simulink model "MotionObjectDetector"  (Simulink 10.0)
settings: Solver=FixedStepAuto  StartTime=0.0  StopTime=inf  RelTol=1e-3  EnableMultiTasking=on
undefined symbols (not defined in the file or in its folder): gray, Horn, hot, iut_dim, Kanade, Lucas, none, num_targets, pfactor, Rec, Schunck, SDTV, strel, target_dim, target_dim_nopyramid, videoinput
libraries: visionsinks x10, visionmorphops x7, visionanalysis x6, visionstatistics x5, visiontransforms x5, visiontextngfix x4, visionconversions x4, dspvision x3, visiongeotforms x2, visionutilities x2, imaqlib x1, visionsources x1
(part 1 of 2)
settings Model: Creator=fredd  LastModifiedBy=fredd  SimulationMode=accelerator  OrderedModelArguments=off
settings SolverCC: PositivePriorityOrder=on  AutoInsertRateTranBlk=on
settings DataIOCC: SaveFormat=Dataset  ReturnWorkspaceOutputs=on
settings OptimizationCC: DefaultParameterBehavior=Inlined  EnhancedBackFolding=on  PassReuseOutputArgsAs=Individual arguments  ZeroExternalMemoryAtStartup=off  ZeroInternalMemoryAtStartup=off  LifeSpan=auto  MaxStackSize=64  OptimizeBlockOrder=speed  DifferentSizesBufferReuse=on  OptimizationCustomize=off  EfficientTunableParamExpr=on
settings DebuggingCC: UnderspecifiedInitializationDetection=Simplified  MergeDetectMultiDrivingBlocksExec=error  ParameterTunabilityLossMsg=error  SFUnexpectedBacktrackingDiag=error  SFNoUnconditionalDefaultTransitionDiag=error  SFExecutionAtInitializationDiag=warning  ArithmeticOperatorsInVariantConditions=error
settings HardwareCC: ProdLargestAtomicInteger=Long  ProdLargestAtomicFloat=Double  ProdIntDivRoundTo=Zero  ProdEndianess=LittleEndian  ProdLongLongMode=on  ProdHWDeviceType=ARM Compatible->ARM Cortex
settings ModelReferenceCC: PropagateSignalLabelsOutOfModel=on
settings SFSimCC: SimUseLocalCustomCode=on  CustomCodeUndefinedFunction=FilterOut
settings RTWCC: Description=Embedded Coder  SystemTargetFile=ert.tlc  TemplateMakefile=ert_default_tmf  GenerateReport=on  RTWUseLocalCustomCode=on  Toolchain=GNU GCC Raspberry Pi  BuildConfiguration=Faster Runs  IncludeHyperlinkInReport=on  LaunchReport=on  GenerateTraceInfo=on  GenerateTraceReport=on  GenerateTraceReportSl=on  GenerateTraceReportSf=on  GenerateTraceReportEml=on
settings CodeAppCC: ForceParamTrailComments=on  IgnoreCustomStorageClasses=off  OperatorAnnotations=on  SimulinkDataObjDesc=on  SFDataObjDesc=on  InsertBlockDesc=on  StateflowObjectComments=off
settings ERTTargetCC: SupportVariableSizeSignals=on  ERTCustomFileTemplate=example_file_process.tlc
settings ConfigComp: CovMetricSettings=dwe  CovHtmlReporting=off  CovSaveCumulativeToWorkspaceVar=off  CovSaveSingleToWorkspaceVar=off

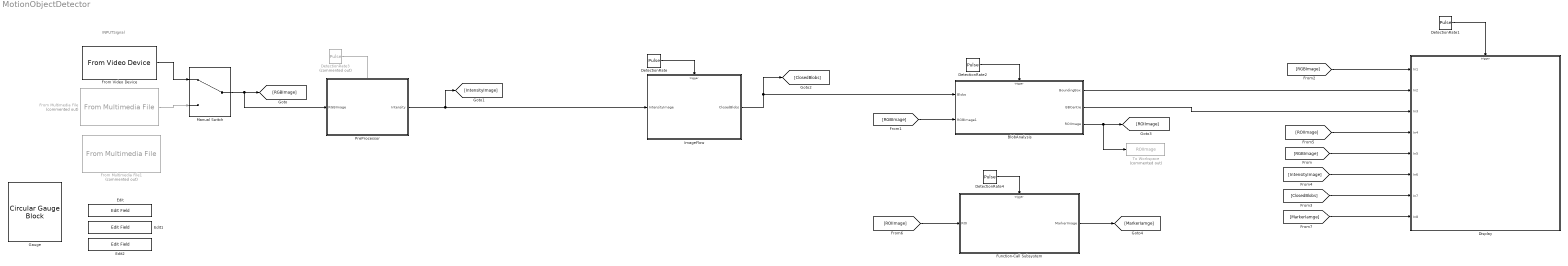
== system MotionObjectDetector ==
  note: INPUTSignal
  BlobAnalysis : Subsystem
  DetectionRate : DiscretePulseGenerator  PulseType=Time based  Period=1/15  PulseWidth=5
  DetectionRate1 : DiscretePulseGenerator  PulseType=Time based  Period=1/30  PulseWidth=5
  DetectionRate2 : DiscretePulseGenerator  PulseType=Time based  Period=1/5  PulseWidth=5
  DetectionRate3 : DiscretePulseGenerator  Commented=on  PulseType=Time based  Period=1/50  PulseWidth=5
  DetectionRate4 : DiscretePulseGenerator  PulseType=Time based  Period=1/2  PulseWidth=5
  Display : Subsystem
  Edit : EditField  LabelPosition=Hide  ShowInitialText=on  Alignment=Center
  Edit1 : EditField  LabelPosition=Hide  ShowInitialText=on  Alignment=Center
  Edit2 : EditField  LabelPosition=Hide  ShowInitialText=on  Alignment=Center
  From Multimedia File : dspvision/From Multimedia File  Commented=on  inputFilename=D:\Documents\GitHub\E-ProjectDocs\CrabDetection\RedCrabVideo2.mp4  readRange=[1 Inf]  loop=on  numPlays=inf  outputStreams=Video only  videoDataType=single  audioDataType=int16  inheritSampleTime=on  userDefinedSampleTime=1/30  noAudioOutput=off  isIntensityVideo=off  fourcc=RGB  colorVideoFormat=One multidimensional signal  outputEOF=off  dataOrg=Column-major  audioFrameSize=1024  computeAudioFrameSize=off  outSamplingMode=Sample based
      settings: SourceProductName=DSP System Toolbox  SourceProductBaseCode=DS
  From Multimedia File1 : dspvision/From Multimedia File  Commented=on  inputFilename=D:\Documents\GitHub\E-ProjectDocs\CrabDetection\RedCrabVideo2.mp4  readRange=[1 Inf]  loop=on  numPlays=inf  outputStreams=Video only  videoDataType=single  audioDataType=int16  inheritSampleTime=on  userDefinedSampleTime=1/30  noAudioOutput=off  isIntensityVideo=off  fourcc=RGB  colorVideoFormat=One multidimensional signal  outputEOF=off  dataOrg=Column-major  audioFrameSize=1024  computeAudioFrameSize=off  outSamplingMode=Sample based
      settings: SourceProductName=DSP System Toolbox  SourceProductBaseCode=DS
  From Video Device : imaqlib/From Video Device  DeviceMenu=winvideo 1 (HD Pro Webcam C920)  Device=winvideo 1 (HD Pro Webcam C920)  ObjConstructor=videoinput('winvideo', 1)  VideoFormatMenu=MJPG_1280x720  VideoFormat=MJPG_1280x720  VideoSource=input1  ROIPosition=[0 0 720 1280]  EnableHWTrigger=off  TriggerConfiguration=none/none  SampleTime=1/30  OutputPortsMode=One multidimensional signal  DataType=single  CanDoHWTrigger=no  ReturnedColorSpace=rgb  BlockHandle=4612.0004  ROIWidth=1280  ROIHeight=720  ROIColumn=0  ROIRow=0  EngXMLPath=C:\Program Files\MATLAB\R2019b\toolbox\imaq\imaq\private  DevXMLPath=C:\ProgramData\MATLAB\SupportPackages\R2019b\toolbox\imaq\supportpackages\genericvideo\adaptor\win64  EngLibPath=C:\Program Files\MATLAB\R2019b\toolbox\imaq\imaqblks\imaqmex\win64  ColorSpace=rgb  BayerSensorAlignment=grbg  ImaqMode=off
      settings: SourceProductName=Image Acquisition Toolbox
  Function-Call Subsystem : Subsystem  TreatAsAtomicUnit=on
  Gauge : CircularGaugeBlock
  ImageFlow : Subsystem
  Manual Switch : ManualSwitch
  PreProcessor : Subsystem
  To Workspace : ToWorkspace  Commented=on  VariableName=ROIImage  SaveFormat=Timeseries  SampleTime=-1
  wires:
  [ROIImage] -> Display/4(In4)
  DetectionRate/1 -> ImageFlow/Trigger
  DetectionRate1/1 -> Display/Trigger
  From Video Device/1 -> Manual Switch/1
  DetectionRate2/1 -> BlobAnalysis/Trigger
  DetectionRate3/1 -> ?
  Manual Switch/1 -> [RGBImage], PreProcessor/1(RGBImage)
  BlobAnalysis/2(BBCentre) -> Display/3(In3)
  BlobAnalysis/1(BoundingBox) -> Display/2(In2)
  ImageFlow/1(ClosedBlobs) -> BlobAnalysis/1(Blobs), [ClosedBlobs]
  [RGBImage] -> BlobAnalysis/2(RGBImage1)
  PreProcessor/1(Intensity) -> ImageFlow/1(IntensityImage), [IntensityImage]
  [RGBImage] -> Display/5(In5)
  [IntensityImage] -> Display/6(In6)
  [ClosedBlobs] -> Display/7(In7)
  [RGBImage] -> Display/1(In1)
  BlobAnalysis/3(ROIImage) -> To Workspace/1, [ROIImage]
  DetectionRate4/1 -> Function-Call Subsystem/Trigger
  [ROIImage] -> Function-Call Subsystem/1(ROI)
  Function-Call Subsystem/1(MarkerImage) -> [MarkerIamge]
  [MarkerIamge] -> Display/8(In8)
  From Multimedia File/1 -> Manual Switch/2

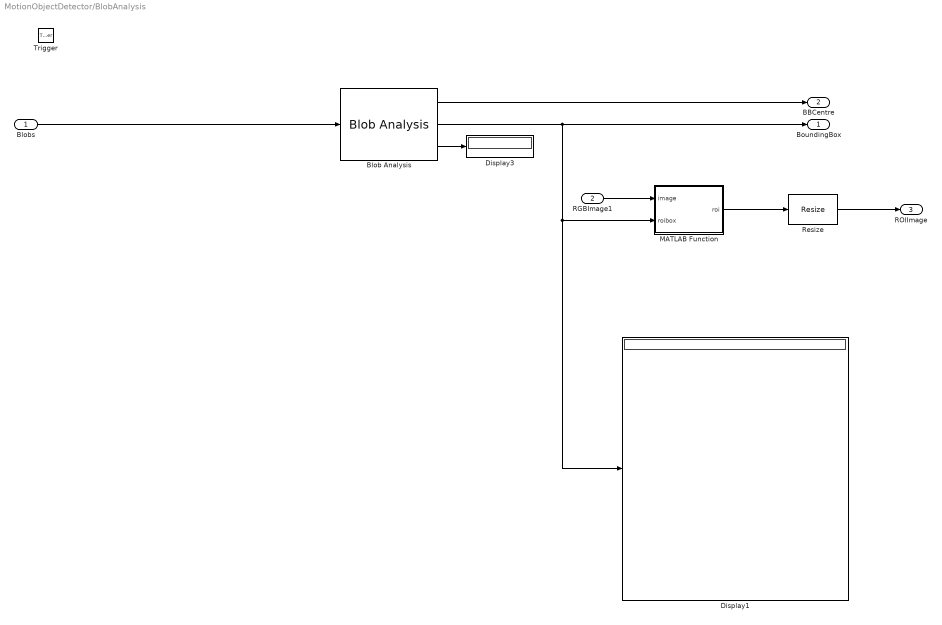
== system MotionObjectDetector/BlobAnalysis ==
  Blobs : Inport
  RGBImage1 : Inport  Port=2
  Trigger : TriggerPort  TriggerType=falling  VariantControl=Variant  PortDimensions=1
  Blob Analysis : visionstatistics/Blob Analysis  Tag=vipblks_row_conv  area=off  centroid=on  bBox=on  majorAxis=off  minorAxis=off  angle=off  eccentricity=off  equivDiameterSq=off  extent=off  perimeter=off  outDT=double  conn=8  isLabel=off  maxBlobs=50  warnIfNumBlobsExceeded=on  isCount=on  useMinArea=on  minArea=1000  useMaxArea=on  maxArea=50000  excludeBorderBlob=off  isOutVarDim=off  isFill=on  fillValues=-1  roundingMode=Floor  overflowMode=off  prodOutputMode=Binary point scaling  prodOutputWordLength=32  prodOutputFracLength=16  prodOutputSlope=2^-16  accumMode=Binary point scaling  accumWordLength=32  accumFracLength=0  accumSlope=2^0  outputMode=Binary point scaling  outputWordLength=32  outputFracLength=16  outputSlope=2^-16  memorySlope=2^-16  firstCoeffMode=Binary point scaling  firstCoeffWordLength=16  firstCoeffFracLength=14  firstCoeffSlope=2^-14  secondCoeffMode=Binary point scaling  secondCoeffWordLength=32  secondCoeffFracLength=16  secondCoeffSlope=2^-16
      settings: SourceProductName=Computer Vision Toolbox
  Display1 : Display
  Display3 : Display
  MATLAB Function : MATLAB Function  TreatAsAtomicUnit=on
  Resize : visiongeotforms/Resize  specify=Number of output rows and columns  rfactor=[500 500]  outCols=25  outRows=25  outRowsCols=[500 500]  interp_method=Bilinear  antialias=on  useROI=off  roiFlag=off  roundingMode=Nearest  overflowMode=on  prodOutputMode=Binary point scaling  prodOutputWordLength=32  prodOutputFracLength=10  prodOutputSlope=2^-10  accumSlope=2^-10  outputSlope=2^-10
      settings: SourceProductName=Computer Vision Toolbox  SourceProductBaseCode=VP
  BoundingBox : Outport
  BBCentre : Outport  Port=2
  ROIImage : Outport  Port=3  InitialOutput=single(zeros(500,500,3))
  wires:
  Blob Analysis/3 -> Display3/1
  RGBImage1/1 -> MATLAB Function/1(image)
  Blobs/1 -> Blob Analysis/1
  Blob Analysis/1 -> BBCentre/1
  MATLAB Function/1(roi) -> Resize/1
  Resize/1 -> ROIImage/1
  Blob Analysis/2 -> MATLAB Function/2(roibox), Display1/1, BoundingBox/1

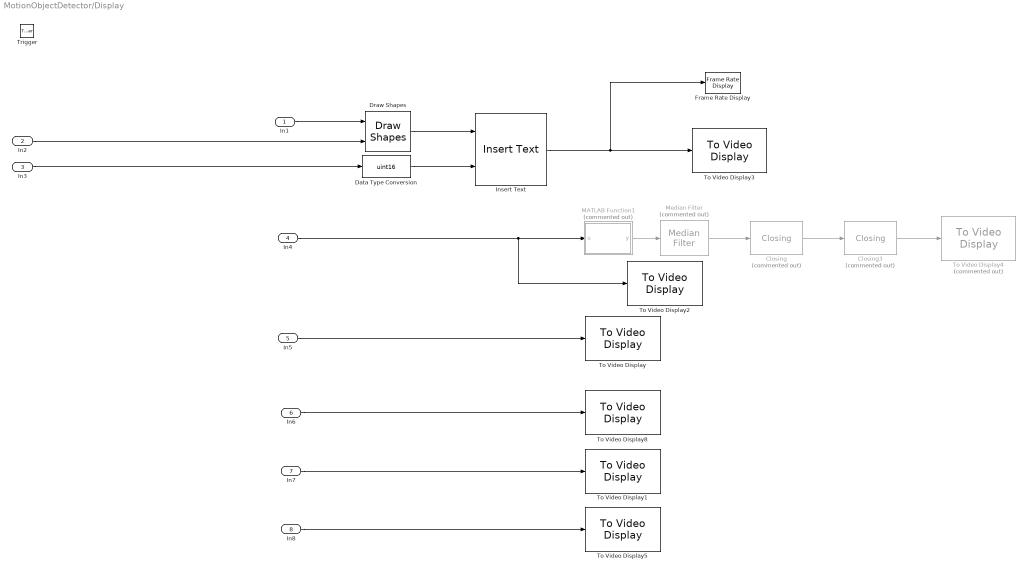
== system MotionObjectDetector/Display ==
  In1 : Inport
  In2 : Inport  Port=2
  In3 : Inport  Port=3
  In4 : Inport  Port=4
  In5 : Inport  Port=5
  In6 : Inport  Port=6
  In7 : Inport  Port=7
  In8 : Inport  Port=8
  Trigger : TriggerPort  TriggerType=falling  VariantControl=Variant  PortDimensions=1
  Closing : visionmorphops/Closing  Commented=on  nhoodsrc=Specify via dialog  strel=strel('rectangle',[60,60])
      settings: SourceProductName=Computer Vision Toolbox  SourceProductBaseCode=VP
  Closing3 : visionmorphops/Closing  Commented=on  nhoodsrc=Specify via dialog  strel=strel('disk',4,4)
      settings: SourceProductName=Computer Vision Toolbox  SourceProductBaseCode=VP
  Data Type Conversion : DataTypeConversion  OutDataTypeStr=uint16
  Draw Shapes : visiontextngfix/Draw Shapes  shape=Rectangles  fill=off  lineWidth=1  fillClrSource=Specify via dialog  display=User-specified value  intensity=200  color=[0 1 0]  opacity=0.6  viewport=Entire image  antialiasing=off  inType=Obsolete  imagePorts=One multidimensional signal  roundingMode=Floor  overflowMode=off  memoryMode=Specify word length  memoryWordLength=16  prodOutputMode=Binary point scaling  prodOutputWordLength=32  prodOutputFracLength=14  prodOutputSlope=2^-14  accumSlope=2^-14  memoryFracLength=15
      settings: SourceProductName=Computer Vision Toolbox
  Frame Rate Display : visionsinks/Frame Rate Display  UpdateRate=10
      settings: SourceProductName=Computer Vision Toolbox  SourceProductBaseCode=VP
  Insert Text : visiontextngfix/Insert Text  inputType=Obsolete  theText='Item'  getTextLocFrom=Input port  textLoc=[1 1]  getTextColorFrom=Specify via dialog  textColor=[0 255 0]  getTextIntensityFrom=Specify via dialog  textIntensity=0  getTextOpacityFrom=Specify via dialog  textOpacity=1.0  dummyVar2=0  dummyVar3=0  dummyVar4=0  imagePorts=One multidimensional signal  isInputTransposed=off  fontFace=LucidaSansRegular  dummyVar1=0  blockFontSize=12  antiAliased=on
      settings: SourceProductName=Computer Vision Toolbox  SourceProductBaseCode=VP
  MATLAB Function1 : MATLAB Function  Commented=on  TreatAsAtomicUnit=on
  Median Filter : visionanalysis/Median Filter  Commented=on  nghbood=[3 3]  outSize=Same as input port I  padType=Circular  padSrc=Specify via dialog  padVal=0  roundingMode=Floor  overflowMode=off  prodOutputSlope=2^-30  accumSlope=2^-30  outputSlope=2^-15
      settings: SourceProductName=Computer Vision Toolbox  SourceProductBaseCode=VP
  To Video Display : visionsinks/To Video Display  windowSizeMode=Normal  openAtMdlStart=on  fullScreen=off  videoWindowX=145  videoWindowY=272  saveWindowSize=off  videoWindowWidth=640  videoWindowHeight=352  inputColorFormat=RGB  inputType=Obsolete  imagePorts=One multidimensional signal  OutputDevice=On-screen video monitor  dataOrg=Column-major  isWindowOpen=off
      settings: SourceProductName=Computer Vision Toolbox
  To Video Display1 : visionsinks/To Video Display  windowSizeMode=Normal  openAtMdlStart=on  fullScreen=off  videoWindowX=1425  videoWindowY=368  saveWindowSize=off  videoWindowWidth=431  videoWindowHeight=259  inputColorFormat=RGB  inputType=Obsolete  imagePorts=One multidimensional signal  OutputDevice=On-screen video monitor  dataOrg=Column-major  isWindowOpen=off
      settings: SourceProductName=Computer Vision Toolbox
  To Video Display2 : visionsinks/To Video Display  windowSizeMode=Normal  openAtMdlStart=on  fullScreen=off  videoWindowX=1085  videoWindowY=363  saveWindowSize=off  videoWindowWidth=328  videoWindowHeight=259  inputColorFormat=RGB  inputType=Obsolete  imagePorts=One multidimensional signal  OutputDevice=On-screen video monitor  dataOrg=Column-major  isWindowOpen=off
      settings: SourceProductName=Computer Vision Toolbox
  To Video Display3 : visionsinks/To Video Display  windowSizeMode=Normal  openAtMdlStart=on  fullScreen=off  videoWindowX=150  videoWindowY=134  saveWindowSize=off  videoWindowWidth=902  videoWindowHeight=488  inputColorFormat=RGB  inputType=Obsolete  imagePorts=One multidimensional signal  OutputDevice=On-screen video monitor  dataOrg=Column-major  isWindowOpen=off
      settings: SourceProductName=Computer Vision Toolbox
  To Video Display4 : visionsinks/To Video Display  Commented=on  windowSizeMode=Normal  openAtMdlStart=on  fullScreen=off  videoWindowX=599  videoWindowY=389  saveWindowSize=off  videoWindowWidth=267  videoWindowHeight=235  inputColorFormat=RGB  inputType=Obsolete  imagePorts=One multidimensional signal  OutputDevice=On-screen video monitor  dataOrg=Column-major  isWindowOpen=off
      settings: SourceProductName=Computer Vision Toolbox
  To Video Display5 : visionsinks/To Video Display  windowSizeMode=Normal  openAtMdlStart=on  fullScreen=off  videoWindowX=1422  videoWindowY=363  saveWindowSize=off  videoWindowWidth=301  videoWindowHeight=259  inputColorFormat=RGB  inputType=Obsolete  imagePorts=One multidimensional signal  OutputDevice=On-screen video monitor  dataOrg=Column-major  isWindowOpen=off
      settings: SourceProductName=Computer Vision Toolbox
  To Video Display8 : visionsinks/To Video Display  windowSizeMode=Normal  openAtMdlStart=on  fullScreen=off  videoWindowX=1093  videoWindowY=79  saveWindowSize=off  videoWindowWidth=350  videoWindowHeight=259  inputColorFormat=RGB  inputType=Obsolete  imagePorts=One multidimensional signal  OutputDevice=On-screen video monitor  dataOrg=Column-major  isWindowOpen=off
      settings: SourceProductName=Computer Vision Toolbox
  wires:
  In5/1 -> To Video Display/1
  Insert Text/1 -> Frame Rate Display/1, To Video Display3/1
  In6/1 -> To Video Display8/1
  In3/1 -> Data Type Conversion/1
  Draw Shapes/1 -> Insert Text/1
  In2/1 -> Draw Shapes/2
  Data Type Conversion/1 -> Insert Text/2
  In1/1 -> Draw Shapes/1
  In7/1 -> To Video Display1/1
  In4/1 -> MATLAB Function1/1(u), To Video Display2/1
  MATLAB Function1/1(y) -> Median Filter/1
  Median Filter/1 -> Closing/1
  Closing/1 -> Closing3/1
  Closing3/1 -> To Video Display4/1
  In8/1 -> To Video Display5/1

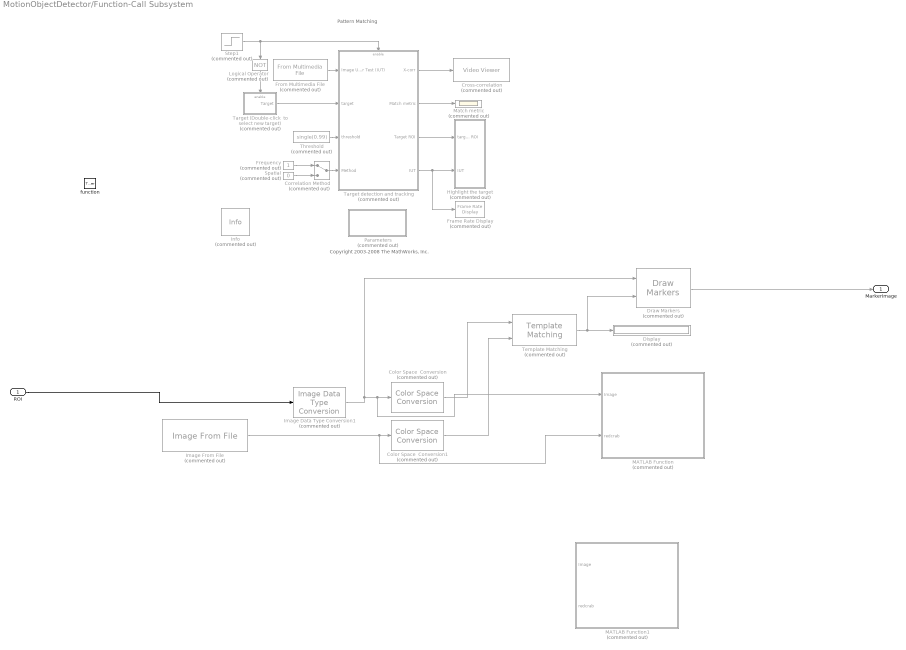
== system MotionObjectDetector/Function-Call Subsystem ==
  note: Pattern Matching
  note: Copyright 2003-2008 The MathWorks, Inc.
  ROI : Inport
  function : TriggerPort  VariantControl=Variant
  Color Space  Conversion : visionconversions/Color Space  Conversion  Commented=on  conversion=Obsolete  conversionActive=R'G'B' to intensity  wp_str=D65  rec=Rec. 601 (SDTV)  sys=1125/60/2:1  imagePorts=One multidimensional signal
  Color Space  Conversion1 : visionconversions/Color Space  Conversion  Commented=on  conversion=Obsolete  conversionActive=R'G'B' to intensity  wp_str=D65  rec=Rec. 601 (SDTV)  sys=1125/60/2:1  imagePorts=One multidimensional signal
  Correlation Method : ManualSwitch  Commented=on
  Cross-correlation : VideoViewer  Commented=on  useColorMap=on  colormapValue=hot(256)  specRange=on  minInputVal=0.9  maxInputVal=0.999  FigPos=[632 384 339 256]
  Display : Display  Commented=on
  Draw Markers : visiontextngfix/Draw Markers  Commented=on  shape=Circle  size=100  fill=off  fillClrSource=Specify via dialog  display=User-specified value  intensity=200  color=[0 255 0]  opacity=0.6  viewport=Entire image  antialiasing=off  inType=Obsolete  imagePorts=One multidimensional signal  roundingMode=Floor  overflowMode=off  memoryMode=Specify word length  memoryWordLength=16  memoryFracLength=15  memorySlope=2^-14  prodOutputMode=Binary point scaling  prodOutputWordLength=32  prodOutputFracLength=14  prodOutputSlope=2^-14  accumSlope=2^-14
      settings: SourceProductName=Computer Vision Toolbox  SourceProductBaseCode=VP
  Frame Rate Display : visionsinks/Frame Rate Display  Commented=on  UpdateRate=10
      settings: SourceProductName=Computer Vision Toolbox  SourceProductBaseCode=VP
  Frequency : Constant  Commented=on  VectorParams1D=off
  From Multimedia File : dspvision/From Multimedia File  Commented=on  inputFilename=vipboard.mp4  readRange=[1 Inf]  loop=on  numPlays=inf  outputStreams=Video only  videoDataType=single  audioDataType=int16  inheritSampleTime=on  userDefinedSampleTime=1/30  noAudioOutput=off  isIntensityVideo=off  fourcc=Intensity  colorVideoFormat=Separate color signals  outputEOF=off  dataOrg=Column-major  audioFrameSize=1024  computeAudioFrameSize=off  outSamplingMode=Frame based
      settings: SourceProductName=DSP System Toolbox  SourceProductBaseCode=DS
  Highlight the target : Subsystem  Commented=on
  Image Data Type Conversion1 : visionconversions/Image Data Type Conversion  Commented=on  outDT=uint8  isSigned=on  wordLen=16  numFracBits=0
      settings: SourceProductName=Computer Vision Toolbox  SourceProductBaseCode=VP
  Image From File : visionsources/Image From File  Tag=vipblks_nd  Commented=on  FileName=D:\Documents\GitHub\E-ProjectDocs\CrabDetection\redcrab.jpeg  Ts=inf  imagePorts=One multidimensional signal  OutPortLabels=R|G|B  ImageDataType=Inherit from input image  sdImageDataType=uint(8)  Signed=on  WordLength=16  FractionLengthMode=User-defined  FractionLength=15
      settings: SourceProductName=Computer Vision Toolbox
  Info : vipmisc/Info  Commented=on  SystemSampleTime=-1  Latency=0  AutoFrameSizeCalculation=off
      settings: SourceProductName=Computer Vision Toolbox  SourceProductBaseCode=VP
  Logical Operator : Logic  Commented=on  Operator=NOT  AllPortsSameDT=off  OutDataTypeStr=boolean
  MATLAB Function : MATLAB Function  Commented=on  TreatAsAtomicUnit=on
  MATLAB Function1 : MATLAB Function  Commented=on  TreatAsAtomicUnit=on
  Match metric : Scope  Commented=on
  Parameters : Subsystem  Commented=on  mask(Pyramiding factor){pfactor=2, num_targets=2, target=[90 99 80 66 86 90 80 69 56 57 57 59 63 63 63 63 62 62 62 62 62 62 61 61 59 59 59 58 57 57 56 56 56 55 56 56 57 57 58 58 58 59 59 59 59 58 58 58 57 57 57 57 58 61 65 67 67 67 67 66 66 66 67 67 67 67 97;102 98 112 114 98 77 79 70 66 72 72 74 79 80 80 80 79 79 79 79 78 76 72 70 70 70 71 72 73 73 74 74 76 76 77 77 78 78 79 79 79 80 80 80 80 80 81 81 81 81 81 81 83 85 86 88 88 86 80 78 78 78 78 79 79 79 97;86 100 101 107 99 81 83 73 72 79 72 74 78 79 79 79 74 72 72 72 71 71 71 70 69 69 66 66 65 67 71 73 72 70 67 66 66 67 67 66 66 66 66 66 66 66 65 65 64 63 62 61 61 63 64 66 67 67 49 54 61 65 71 76 83 87 98;81 107 101 107 99 83 77 78 72 64 48 45 42 41 40 38 36 33 31 30 30 30 31 31 34 35 37 38 38 38 37 37 37 37 36 35 30 29 30 30 30 31 31 31 30 30 29 29 28 28 28 28 28 28 27 27 27 27 28 36 51 58 72 76 83 87 98;92 105 101 107 98 83 79 76 59 48 31 29 26 24 24 24 24 26 24 23 22 21 20 20 19 19 17 17 19 19 20 20 20 20 21 22 27 30 31 31 31 33 33 33 34 34 35 35 35 36 36 36 36 36 20 20 20 20 17 24 40 48 72 76 83 87 99;100 101 105 107 98 84 86 67 48 49 40 41 44 45 47 48 52 55 55 55 55 56 56 56 56 57 56 56 57 57 58 58 61 63 66 67 65 64 64 63 63 63 63 63 63 63 77 77 76 74 73 72 71 70 70 69 69 69 43 47 55 58 72 76 83 87 99;114 118 111 106 97 85 74 62 54 55 77 84 88 84 90 90 90 90 90 90 88 87 83 81 86 87 87 87 86 86 85 85 85 86 88 90 90 91 90 90 88 88 87 87 86 86 90 90 90 90 90 90 91 91 92 92 93 93 92 65 45 54 70 73 80 85 100;119 120 114 106 95 85 74 62 54 57 77 84 88 84 90 90 90 90 90 90 88 87 83 81 86 87 87 87 87 87 86 86 87 88 88 90 90 91 90 90 88 88 87 87 86 86 90 90 90 90 90 90 91 91 92 92 93 93 92 65 45 54 70 73 80 85 100;116 116 114 106 97 87 74 63 55 57 77 84 88 84 88 88 88 88 88 88 87 86 83 81 86 87 87 87 87 87 88 88 90 88 90 90 90 90 90 90 88 88 87 87 86 86 88 88 88 88 90 90 90 90 91 91 92 92 91 66 47 52 69 72 80 86 99;115 115 113 106 97 88 74 64 56 57 77 84 88 84 86 86 87 87 87 88 87 86 83 81 86 87 87 86 86 87 88 90 90 90 90 90 90 90 90 90 88 88 87 87 86 86 88 88 88 88 90 90 90 90 91 91 92 92 88 69 49 50 69 72 81 86 99;115 115 114 107 98 92 74 65 57 57 77 84 88 84 85 85 85 86 86 86 86 85 83 81 86 86 86 86 86 86 88 88 88 90 88 88 90 90 90 90 88 88 88 87 87 87 88 88 88 88 88 88 90 90 90 90 90 90 87 71 51 49 67 72 81 87 99;115 115 115 108 98 92 74 66 58 57 77 84 88 84 83 83 84 85 85 86 86 85 83 81 86 86 86 85 85 85 87 87 87 88 88 88 88 88 90 90 88 88 88 87 87 87 87 87 87 87 88 88 88 88 90 90 90 90 85 73 54 47 67 71 81 87 98;115 115 120 111 98 87 76 67 59 57 76 83 87 83 83 83 84 85 85 86 86 85 84 81 85 85 85 85 85 85 86 86 86 87 87 87 87 87 88 88 87 87 87 86 86 86 86 86 86 86 87 87 87 87 88 88 88 88 84 73 54 45 66 71 81 87 98;115 115 120 112 98 86 77 70 59 57 74 81 86 81 83 83 84 84 85 85 85 85 84 83 84 84 85 85 85 85 86 86 86 87 87 87 87 87 88 87 87 87 87 86 86 86 86 86 86 86 87 87 87 87 87 87 87 87 83 73 54 44 66 71 83 88 98;115 115 118 113 98 85 79 70 61 56 73 80 85 80 84 84 84 85 85 86 86 85 85 83 83 83 84 85 85 85 86 86 86 86 86 86 86 86 86 86 85 85 85 85 85 85 86 86 86 86 86 86 86 86 86 86 86 86 83 73 54 44 66 71 83 88 98;115 115 116 113 99 86 80 71 61 56 72 79 84 79 84 84 84 85 85 86 86 85 85 83 81 81 84 85 85 85 85 86 86 86 86 86 86 86 86 85 85 85 85 85 85 85 85 85 85 85 86 86 86 86 86 86 86 86 81 72 52 43 66 71 83 88 98;114 114 115 113 100 87 80 71 61 56 71 78 83 78 84 84 84 85 85 85 85 85 85 83 81 81 84 84 85 85 85 85 85 85 85 85 85 85 85 85 85 85 85 85 85 85 85 85 85 85 85 85 85 85 85 85 85 85 81 72 52 43 65 70 81 87 98;114 115 114 113 101 88 81 72 61 56 71 78 83 78 85 85 85 85 85 85 85 85 83 80 81 83 84 84 85 85 85 85 85 85 85 85 85 85 85 84 84 84 84 84 84 84 85 85 85 85 85 85 85 85 85 85 85 85 81 72 52 43 65 70 81 87 98;114 113 113 112 101 88 81 72 61 56 71 78 83 78 85 85 85 85 85 85 84 83 78 79 83 83 84 84 84 84 84 85 85 85 85 85 84 84 85 85 85 85 85 85 85 85 85 85 85 85 85 85 85 85 85 85 85 85 81 72 52 43 65 70 81 87 98;112 111 111 111 101 88 81 72 61 56 71 78 83 78 85 85 85 85 84 84 84 83 76 77 83 84 84 84 84 84 84 84 84 84 ...(+7884 chars)], targetBBox=[35 171 66.0000000000001 56]}
      mask prompts: pfactor "Pyramiding factor:"; num_targets "Number of similar targets to detect:"; targetBBox "Target bounding box:"
      mask help: The pyramiding factor is used to scale the input video so that the cross-correlation is performed on a much smaller video frame thus speeding up the pattern matching process. The factor can be any number from 1 to 5. The accuracy of the match will degrade proportionately to the size of the pyramiding factor.
      mask init:
      | if num_targets <= 0
      |     error('Number of targets must be greater than 0');
      | end
      mask TypeOptions pfactor: 0 | 1 | 2 | 3 | 4 | 5
      mask Display: disp('Edit\nParameters')
  Spatial : Constant  Commented=on  Value=0  VectorParams1D=off
  Step1 : Step  Commented=on  Time=eps
  Target (Double-click  to select new target) : Subsystem  Commented=on
      mask init:
      | model_path = [get(bdroot(gcbh),'Path'), '/Parameters'];
      | target_img = uint8(eval(get_param(model_path,'target')));
      settings: OpenFcn=vippattern_gettemplate
      mask Display: image(repmat(target_img,[1,1,3]))
  Target detection and tracking : Subsystem  Commented=on
  Template Matching : visionanalysis/Template Matching  Commented=on  metric=Sum of absolute differences  output=Best match location  method=Three-step  nMetric=off  nSize=3  roi=off  roiValid=on  roundingMode=Floor  overflowMode=off  prodOutputMode=Binary point scaling  prodOutputWordLength=32  prodOutputFracLength=0  prodOutputSlope=2^0  accumMode=Binary point scaling  accumWordLength=32  accumFracLength=0  accumSlope=2^0  outputSlope=2^0
      settings: SourceProductName=Computer Vision Toolbox  SourceProductBaseCode=VP
  Threshold : Constant  Commented=on  Value=single(0.99)  VectorParams1D=off
  MarkerImage : Outport
  wires:
  Template Matching/1 -> Display/1, Draw Markers/2
  Color Space  Conversion/1 -> Template Matching/1
  Color Space  Conversion1/1 -> Template Matching/2
  Image From File/1 -> MATLAB Function/2(redcrab), Color Space  Conversion1/1
  Draw Markers/1 -> MarkerImage/1
  Image Data Type Conversion1/1 -> Draw Markers/1, MATLAB Function/1(Image), Color Space  Conversion/1
  ROI/1 -> Image Data Type Conversion1/1
  Spatial/1 -> Correlation Method/2
  Target (Double-click  to select new target)/1(Target) -> Target detection and tracking/2(target)
  Target detection and tracking/3(Target ROI) -> Highlight the target/1(target ROI)
  Threshold/1 -> Target detection and tracking/3(threshold)
  Target detection and tracking/1(X-corr) -> Cross-correlation/1
  From Multimedia File/1 -> Target detection and tracking/1(Image Under Test (IUT))
  Step1/1 -> Target detection and tracking/Enable, Logical Operator/1
  Target detection and tracking/2(Match metric) -> Match metric/1
  Logical Operator/1 -> Target (Double-click  to select new target)/Enable
  Correlation Method/1 -> Target detection and tracking/4(Method)
  Frequency/1 -> Correlation Method/1
  Target detection and tracking/4(IUT) -> Highlight the target/2(IUT), Frame Rate Display/1

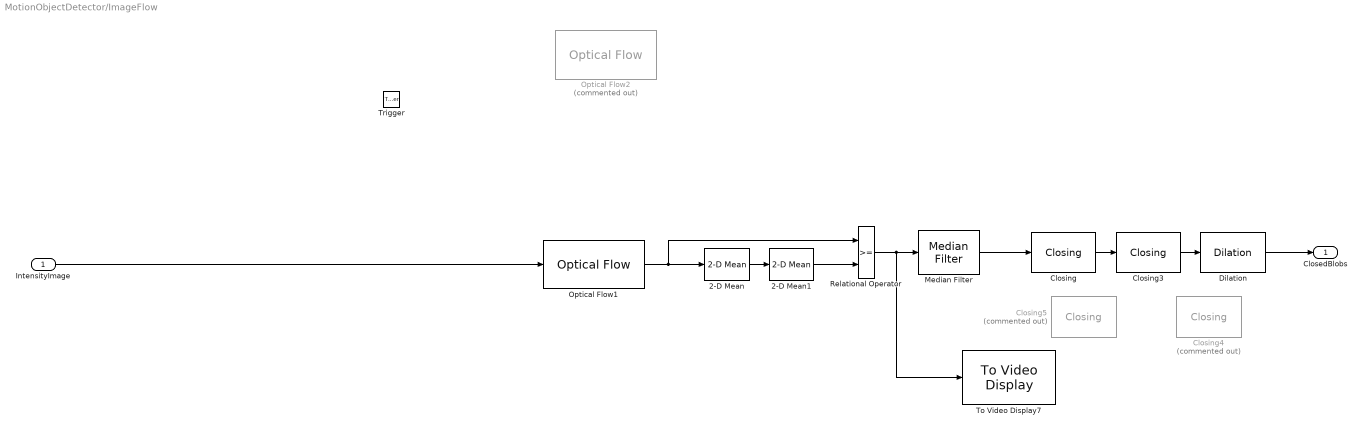
== system MotionObjectDetector/ImageFlow ==
  IntensityImage : Inport
  Trigger : TriggerPort  TriggerType=falling  VariantControl=Variant  PortDimensions=1
  2-D Mean : visionstatistics/2-D Mean  run=off  reset_popup=None  directionMode=Entire input  dimension=1  treatSBRowAsCol=on  outputLastDataTypeStr=Inherit: Same as accumulator  accumMode=Binary point scaling  accumWordLength=32  accumFracLength=0  accumLastDataTypeStr=fixdt([],32,0)  roiEnable=off  roiType=Rectangles  roiPortion=Entire ROI  roiOutput=Individual statistics for each ROI  roiFlag=off  roundingMode=Floor  overflowMode=off  accumDataTypeStr=fixdt([],32,0)  outputDataTypeStr=Inherit: Same as accumulator  outputMin=[]  outputMax=[]
      settings: SourceProductName=Computer Vision Toolbox  SourceProductBaseCode=VP
  2-D Mean1 : visionstatistics/2-D Mean  run=on  reset_popup=None  directionMode=Entire input  dimension=1  treatSBRowAsCol=on  outputLastDataTypeStr=Inherit: Same as accumulator  accumMode=Binary point scaling  accumWordLength=32  accumFracLength=0  accumLastDataTypeStr=fixdt([],32,0)  roiEnable=off  roiType=Rectangles  roiPortion=Entire ROI  roiOutput=Individual statistics for each ROI  roiFlag=off  roundingMode=Floor  overflowMode=off  accumDataTypeStr=fixdt([],32,0)  outputDataTypeStr=Inherit: Same as accumulator  outputMin=[]  outputMax=[]
      settings: SourceProductName=Computer Vision Toolbox  SourceProductBaseCode=VP
  Closing : visionmorphops/Closing  nhoodsrc=Specify via dialog  strel=strel('rectangle',[60,60])
      settings: SourceProductName=Computer Vision Toolbox  SourceProductBaseCode=VP
  Closing3 : visionmorphops/Closing  nhoodsrc=Specify via dialog  strel=strel('disk',4,4)
      settings: SourceProductName=Computer Vision Toolbox  SourceProductBaseCode=VP
  Closing4 : visionmorphops/Closing  Commented=on  nhoodsrc=Specify via dialog  strel=strel('disk',8,8)
      settings: SourceProductName=Computer Vision Toolbox  SourceProductBaseCode=VP
  Closing5 : visionmorphops/Closing  Commented=on  nhoodsrc=Specify via dialog  strel=strel('rectangle',[5,5])
      settings: SourceProductName=Computer Vision Toolbox  SourceProductBaseCode=VP
  Dilation : visionmorphops/Dilation  nhoodsrc=Specify via dialog  strel=[1 1; 1 1]
      settings: SourceProductName=Computer Vision Toolbox  SourceProductBaseCode=VP
  Median Filter : visionanalysis/Median Filter  nghbood=[3 3]  outSize=Same as input port I  padType=Circular  padSrc=Specify via dialog  padVal=0  roundingMode=Floor  overflowMode=off  prodOutputSlope=2^-30  accumSlope=2^-30  outputSlope=2^-15
      settings: SourceProductName=Computer Vision Toolbox  SourceProductBaseCode=VP
  Optical Flow1 : visionanalysis/Optical Flow  method=Lucas-Kanade  gradMethod=Derivative of Gaussian  which2img=Current frame and N-th frame back  N=34  lambda=1  numInports=7  sigmaS=1  sigmaW=1  discardNormalFlow=off  outputCurrentImage=off  stop_criteria=When maximum number of iterations is reached  maxIter=10  maxAllowAbsDiff=eps  outVelForm=Magnitude-squared  eigTh=0.009  roundingMode=Nearest  overflowMode=on  prodOutputMode=Binary point scaling  prodOutputWordLength=32  prodOutputFracLength=20  prodOutputSlope=2^-20  accumSlope=2^-20  memorySlope=2^-20  firstCoeffSlope=2^-20  outputMode=Binary point scaling  outputWordLength=32  outputFracLength=20  outputSlope=2^-20
      settings: SourceProductName=Computer Vision Toolbox  SourceProductBaseCode=VP
  Optical Flow2 : visionanalysis/Optical Flow  Commented=on  method=Horn-Schunck  gradMethod=Derivative of Gaussian  which2img=Current frame and N-th frame back  N=15  lambda=1  numInports=7  sigmaS=1  sigmaW=1  discardNormalFlow=off  outputCurrentImage=on  stop_criteria=When maximum number of iterations is reached  maxIter=10  maxAllowAbsDiff=eps  outVelForm=Magnitude-squared  eigTh=0.009  roundingMode=Nearest  overflowMode=on  prodOutputMode=Binary point scaling  prodOutputWordLength=32  prodOutputFracLength=20  prodOutputSlope=2^-20  accumSlope=2^-20  memorySlope=2^-20  firstCoeffSlope=2^-20  outputMode=Binary point scaling  outputWordLength=32  outputFracLength=20  outputSlope=2^-20
      settings: SourceProductName=Computer Vision Toolbox  SourceProductBaseCode=VP
  Relational Operator : RelationalOperator  OutDataTypeStr=boolean  RndMeth=Nearest
  To Video Display7 : visionsinks/To Video Display  windowSizeMode=Normal  openAtMdlStart=on  fullScreen=off  videoWindowX=1229  videoWindowY=1171  saveWindowSize=off  videoWindowWidth=434  videoWindowHeight=249  inputColorFormat=RGB  inputType=Obsolete  imagePorts=One multidimensional signal  OutputDevice=On-screen video monitor  dataOrg=Column-major  isWindowOpen=off
      settings: SourceProductName=Computer Vision Toolbox
  ClosedBlobs : Outport
  wires:
  Closing/1 -> Closing3/1
  Relational Operator/1 -> To Video Display7/1, Median Filter/1
  2-D Mean/1 -> 2-D Mean1/1
  2-D Mean1/1 -> Relational Operator/2
  Optical Flow1/1 -> Relational Operator/1, 2-D Mean/1
  IntensityImage/1 -> Optical Flow1/1
  Closing3/1 -> Dilation/1
  Median Filter/1 -> Closing/1
  Dilation/1 -> ClosedBlobs/1

== system MotionObjectDetector/PreProcessor ==
  RGBImage : Inport
  Color Space  Conversion : visionconversions/Color Space  Conversion  conversion=Obsolete  conversionActive=R'G'B' to intensity  wp_str=D65  rec=Rec. 601 (SDTV)  sys=1125/60/2:1  imagePorts=One multidimensional signal
  Contrast Adjustment : visionanalysis/Contrast Adjustment  methodInputRange=Full input data range [min max]  rangeIn=[0 255]  fracSaturate=[1 1]  isBinNum=on  binNum=256  methodOutputRange=Full data type range  rangeOut=[0 255]  roundingMode=Floor  overflowMode=off  prod1Mode=Binary point scaling  prod1WordLength=32  prod1FracLength=16  prod1Slope=2^-16  prod2Mode=Binary point scaling  prod2WordLength=32  prod2FracLength=16  prod2Slope=2^-16
      settings: SourceProductName=Computer Vision Toolbox  SourceProductBaseCode=VP
  Intensity : Outport
  wires:
  RGBImage/1 -> Color Space  Conversion/1
  Contrast Adjustment/1 -> Intensity/1
  Color Space  Conversion/1 -> Contrast Adjustment/1

== system MotionObjectDetector/Function-Call Subsystem/Highlight the target ==
  target ROI : Inport
  IUT : Inport  Port=2
  Convert to RGB : Subsystem
  Draw Shapes : visiontextngfix/Draw Shapes  shape=Rectangles  fill=off  lineWidth=1  fillClrSource=Specify via dialog  display=User-specified value  intensity=200  color=[0 255 0]  opacity=0.6  viewport=Entire image  antialiasing=off  inType=Obsolete  imagePorts=One multidimensional signal  roundingMode=Floor  overflowMode=off  memoryMode=Specify word length  memoryWordLength=16  prodOutputMode=Binary point scaling  prodOutputWordLength=32  prodOutputFracLength=14  prodOutputSlope=2^-14  accumSlope=2^-14  memoryFracLength=15
      settings: SourceProductName=Computer Vision Toolbox
  Overlay the ROI on the target : VideoViewer  colormapValue=gray(256)  FigPos=[255 386 360 262]  trueSizedOnce=on
  wires:
  Draw Shapes/1 -> Overlay the ROI on the target/1
  target ROI/1 -> Draw Shapes/2
  Convert to RGB/1(Image) -> Draw Shapes/1
  IUT/1 -> Convert to RGB/1(I)

== system MotionObjectDetector/Function-Call Subsystem/Parameters ==

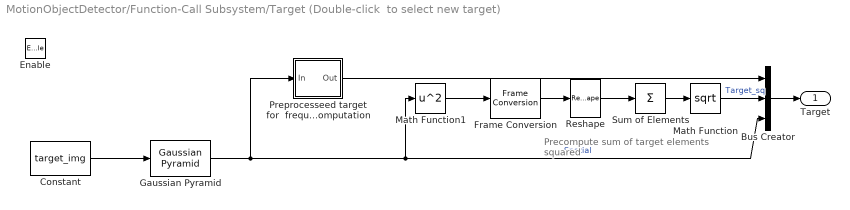
== system MotionObjectDetector/Function-Call Subsystem/Target (Double-click  to select new target) ==
  note: Precompute sum of target elements
      | squared
  Enable : EnablePort  PropagateVarSize=During execution
  Bus Creator : BusCreator  Inputs=3
  Constant : Constant  Value=target_img  VectorParams1D=off  OutDataTypeStr=single
  Frame Conversion : FrameConversion  OutFrame=Sample-based
  Gaussian Pyramid : visiontransforms/Gaussian Pyramid  operation=Reduce  level=pfactor  source="Default separable filter [1/4-a/2  1/4  a  1/4  1/4-a/2]"  a=0.375  coef=[0.0625 0.25 0.375 0.25 0.0625]  hiddenCoef=[1/4-0.375/2 1/4 0.375 1/4 1/4-0.375/2]  roundingMode=Floor  overflowMode=off  firstCoeffMode=Specify word length  firstCoeffWordLength=16  firstCoeffFracLength=16  firstCoeffSlope=2^-16  prodOutputMode=Binary point scaling  prodOutputWordLength=32  prodOutputFracLength=10  prodOutputSlope=2^-10  accumSlope=2^0  outputMode=Binary point scaling  outputWordLength=32  outputFracLength=10  outputSlope=2^-10
      settings: SourceProductName=Computer Vision Toolbox  SourceProductBaseCode=VP
  Math Function : Math  Operator=sqrt  SaturateOnIntegerOverflow=on
  Math Function1 : Math  Operator=square  SaturateOnIntegerOverflow=on
  Preprocesseed target for  frequency domain computation : Subsystem
  Reshape : Reshape
  Sum of Elements : Sum  Inputs=+
  Target : Outport
  wires:
  Preprocesseed target for  frequency domain computation/1(Out) -> Bus Creator/1
  Bus Creator/1 -> Target/1
  Constant/1 -> Gaussian Pyramid/1
  Gaussian Pyramid/1 -> Preprocesseed target for  frequency domain computation/1(In), Bus Creator/3, Math Function1/1  "Spatial"
  Math Function1/1 -> Frame Conversion/1
  Sum of Elements/1 -> Math Function/1
  Reshape/1 -> Sum of Elements/1
  Math Function/1 -> Bus Creator/2  "Target_sq"
  Frame Conversion/1 -> Reshape/1

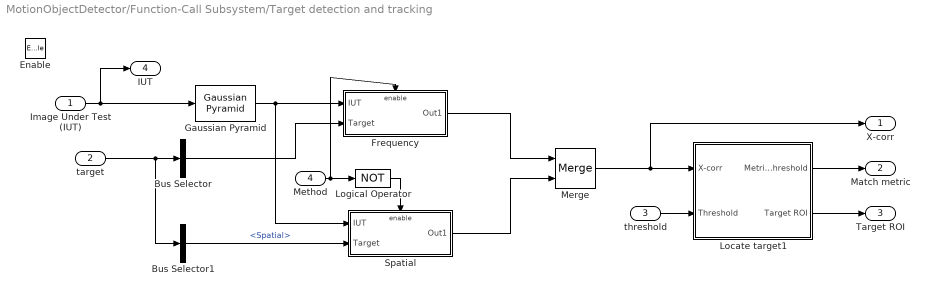
== system MotionObjectDetector/Function-Call Subsystem/Target detection and tracking ==
  Image Under Test (IUT) : Inport
  target : Inport  Port=2
  threshold : Inport  Port=3
  Method : Inport  Port=4
  Enable : EnablePort  PropagateVarSize=During execution
  Bus Selector : BusSelector  OutputSignals=Frequency,Target_sq  OutputAsBus=on
  Bus Selector1 : BusSelector  OutputSignals=Spatial
  Frequency : Subsystem  TreatAsAtomicUnit=on
  Gaussian Pyramid : visiontransforms/Gaussian Pyramid  operation=Reduce  level=pfactor  source="Default separable filter [1/4-a/2  1/4  a  1/4  1/4-a/2]"  a=0.375  coef=[0.0625 0.25 0.375 0.25 0.0625]  hiddenCoef=[1/4-0.375/2 1/4 0.375 1/4 1/4-0.375/2]  roundingMode=Floor  overflowMode=off  firstCoeffMode=Specify word length  firstCoeffWordLength=16  firstCoeffFracLength=16  firstCoeffSlope=2^-16  prodOutputMode=Binary point scaling  prodOutputWordLength=32  prodOutputFracLength=10  prodOutputSlope=2^-10  accumSlope=2^0  outputMode=Binary point scaling  outputWordLength=32  outputFracLength=10  outputSlope=2^-10
      settings: SourceProductName=Computer Vision Toolbox  SourceProductBaseCode=VP
  Locate target1 : Subsystem
  Logical Operator : Logic  Operator=NOT  AllPortsSameDT=off  OutDataTypeStr=boolean
  Merge : Merge
  Spatial : Subsystem  TreatAsAtomicUnit=on
  X-corr : Outport
  Match metric : Outport  Port=2
  Target ROI : Outport  Port=3
  IUT : Outport  Port=4
  wires:
  Image Under Test (IUT)/1 -> IUT/1, Gaussian Pyramid/1
  Locate target1/1(Metric and Threshold) -> Match metric/1
  threshold/1 -> Locate target1/2(Threshold)
  Gaussian Pyramid/1 -> Frequency/1(IUT), Spatial/1(IUT)
  target/1 -> Bus Selector/1, Bus Selector1/1
  Bus Selector/1 -> Frequency/2(Target)
  Bus Selector1/1 -> Spatial/2(Target)  "<Spatial>"
  Spatial/1(Out1) -> Merge/2
  Merge/1 -> X-corr/1, Locate target1/1(X-corr)
  Frequency/1(Out1) -> Merge/1
  Logical Operator/1 -> Spatial/Enable
  Method/1 -> Logical Operator/1, Frequency/Enable
  Locate target1/2(Target ROI) -> Target ROI/1

== system MotionObjectDetector/Function-Call Subsystem/Highlight the target/Convert to RGB ==
  I : Inport
  Matrix Concatenate : Concatenate  NumInputs=3  Mode=Multidimensional array  ConcatenateDimension=3
  Image : Outport
  wires:
  I/1 -> Matrix Concatenate/1, Matrix Concatenate/2, Matrix Concatenate/3
  Matrix Concatenate/1 -> Image/1

== system MotionObjectDetector/Function-Call Subsystem/Target (Double-click  to select new target)/Preprocesseed target for  frequency domain computation ==
  In : Inport
  2-D FFT : visiontransforms/2-D FFT  TableOpt=NEW  TableOptActive=Speed  FFTImplementation=Auto  BitRevOrder=off  SkipNorm=off  firstCoeffLastDataTypeStr=Inherit: Same word length as input  accumLastDataTypeStr=Inherit: Same as product output  roundingMode=Floor  overflowMode=off  firstCoeffDataTypeStr=Inherit: Same word length as input  accumDataTypeStr=Inherit: Same as product output  outputMin=[]  outputMax=[]
      settings: SourceProductName=Computer Vision Toolbox  SourceProductBaseCode=VP
  2-D Pad : visionutilities/Image Pad  method=Constant  valSrc=Specify via dialog  value=0  spec=Output size  rowDirection=Right  outRowsMode=User-specified  rowSize=2  outColSize=2^nextpow2(iut_dim(2)+target_dim(2)+1)  colDirection=Bottom  outColsMode=User-specified  colSize=[2 3]  outRowSize=2^nextpow2(iut_dim(1)+target_dim(1)+1)  trunc_flag=None
      settings: SourceProductName=Computer Vision Toolbox  SourceProductBaseCode=VP
  Rotate : visiongeotforms/Rotate  outSizeR=Expanded to fit rotated input image  src_angle=Specify via dialog  unit_angle=Degrees  angle=single(pi)  maxAngle=pi  dispImage=Center  method=Table lookup  fillVal=0  interpMethod=Bilinear  roundingMode=Nearest  overflowMode=on  firstCoeffSlope=2^-10  prodOutputMode=Binary point scaling  prodOutputWordLength=32  prodOutputFracLength=10  prodOutputSlope=2^-10  accumSlope=2^-10  outputSlope=2^-10
      settings: SourceProductName=Computer Vision Toolbox
  Out : Outport
  wires:
  Rotate/1 -> 2-D Pad/1
  2-D Pad/1 -> 2-D FFT/1
  In/1 -> Rotate/1
  2-D FFT/1 -> Out/1  "Frequency"

== system MotionObjectDetector/Function-Call Subsystem/Target detection and tracking/Frequency ==
  IUT : Inport
  Target : Inport  Port=2
  Enable : EnablePort  PropagateVarSize=During execution
  Normalized X-corr in frequency domain : Subsystem
  Out1 : Outport  InitialOutput=0
  wires:
  Normalized X-corr in frequency domain/1(X-corr) -> Out1/1
  IUT/1 -> Normalized X-corr in frequency domain/1(IUT)
  Target/1 -> Normalized X-corr in frequency domain/2(target)

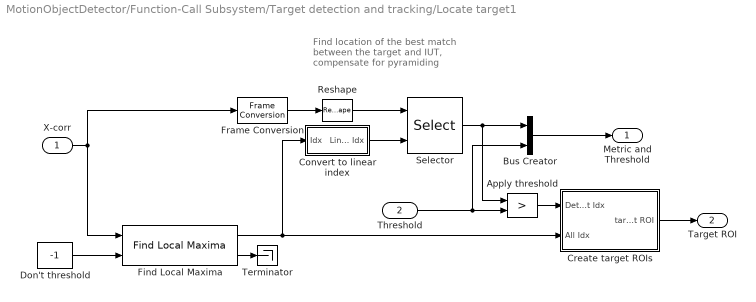
== system MotionObjectDetector/Function-Call Subsystem/Target detection and tracking/Locate target1 ==
  note: Find location of the best match
      | between the target and IUT,
      | compensate for pyramiding
  X-corr : Inport
  Threshold : Inport  Port=2
  Apply threshold : RelationalOperator  Operator=>  OutDataTypeStr=boolean  ZeroCross=off  RndMeth=Nearest
  Bus Creator : BusCreator  Inputs=2
  Convert to linear index : Subsystem
  Create target ROIs : Subsystem
  Don't threshold : Constant  Value=-1  VectorParams1D=off  OutDataTypeStr=Inherit: Inherit via back propagation
  Find Local Maxima : visionstatistics/Find Local Maxima  num_peaks=num_targets  nhood_size=floor(target_dim/2)*2-1  src_thresh=Obsolete9b  src_thresh_inuse=Input port  threshold=10  inputIsHough=off  dt_peak=single  isOutVarDim=off  dt_count=single
      settings: SourceProductName=Computer Vision Toolbox  SourceProductBaseCode=VP
  Frame Conversion : FrameConversion  OutFrame=Sample-based
  Reshape : Reshape
  Selector : Selector  IndexMode=Zero-based  InputPortWidth=prod(((iut_dim-target_dim)+1))  IndexOptions=Index vector (port)  Indices=[1 3]  OutputSizes=1
  Terminator : Terminator
  Metric and Threshold : Outport
  Target ROI : Outport  Port=2
  wires:
  Threshold/1 -> Bus Creator/2, Apply threshold/2
  Create target ROIs/1(target ROI) -> Target ROI/1
  Reshape/1 -> Selector/1
  Convert to linear index/1(Linear Idx) -> Selector/2
  Bus Creator/1 -> Metric and Threshold/1
  Apply threshold/1 -> Create target ROIs/1(Detected-target Idx)
  Don't threshold/1 -> Find Local Maxima/2
  Find Local Maxima/2 -> Terminator/1
  Selector/1 -> Bus Creator/1, Apply threshold/1
  Find Local Maxima/1 -> Create target ROIs/2(All Idx), Convert to linear index/1(Idx)
  X-corr/1 -> Find Local Maxima/1, Frame Conversion/1
  Frame Conversion/1 -> Reshape/1
